simulink model "GoodWe_exec"  (Simulink 3.00)
libraries: execlib x7
settings Model: MaskType=REX sequence  MaskIconFrame=on  MaskIconOpaque=on  MaskIconRotate=none  MaskIconUnits=autoscale

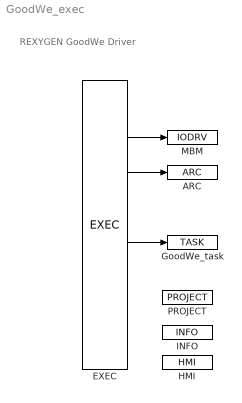
== system GoodWe_exec ==
  note: REXYGEN GoodWe Driver
  ARC : execlib/ARC  atype=3: Disk  asize=102400  nmarks=720  ldaymax=1048576  period=300  timesrc=1: CORETIMER
  EXEC : execlib/EXEC  target=Generic target device  tick=0.01  ntick0=1  ntick1=50  ntick2=100  ntick3=1200  pri0=5  pri1=9  pri2=13  pri3=18  cpu0=-1  cpu1=-1  cpu2=-1  cpu3=-1
  GoodWe_task : execlib/TASK  factor=100  start=0  stop=1  stack=10240  filename=GoodWe_task  MDLOPEN=on
  HMI : execlib/HMI  IncludeHMI=off  HmiDir=hmi  SourceDir=hmisrc  GenerateWebWatch=off  GenerateRexHMI=off  RedirectToHMI=on  Compression=off
  INFO : execlib/INFO  Title=REXYGEN GoodWe Driver  Author=Tomas Cechura  Description=REXYGEN driver for GoodWe Inverters ET series
  MBM : execlib/IODRV  module=MbDrv  classname=MbmDrv  cfgname=GoodWe_RTU_cfg.rio  factor=100  stack=10240  pri=3  timer=off  cpu=-1
  PROJECT : execlib/PROJECT  SourcesOnTarget=on
  wires:
  EXEC/2 -> MBM/1
  EXEC/3 -> ARC/1
  EXEC/5 -> GoodWe_task/1
